simulink model "m03_model_for_state_feedback_design"  (R2021a)
settings: Solver=VariableStepAuto  StartTime=0.0  StopTime=10.0  MaxStep=1e-3  RelTol=1e-3
PreLoadFcn:
  | load feedforward_controller
  | load reduced_model
InitFcn:
  | load feedforward_controller
  | load reduced_model
values from neighbouring files (symbols this model uses):
  U0 = [0 0]    [linearization_data.mat]    (also in linearizedModel_Outputs.mat = [3.61873688012e-10 -3.90256021581e-22])
  Y0 = [0 0]    [linearization_data.mat]    (also in linearizedModel_Outputs.mat = [372.5 36.8372638482])
undefined symbols (not defined in the file or in its folder): X0_red
libraries: acolibjan22 x3
settings Model: Creator=e102261  LastModifiedBy=e102261
settings SolverCC: AlgebraicLoopSolver=TrustRegion
settings DataIOCC: SaveOutput=off  SignalLogging=off  DSMLogging=off  SaveTime=off  ReturnWorkspaceOutputs=off
settings DebuggingCC: ArithmeticOperatorsInVariantConditions=warning
settings SFSimCC: CustomCodeUndefinedFunction=UseInterfaceOnly

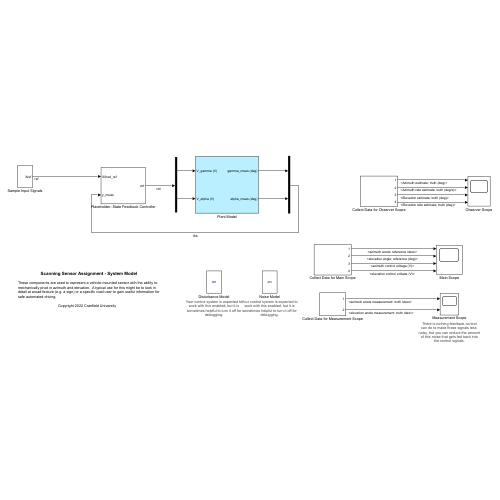
[thumbnail: Simulink's stored preview of the top-level diagram]
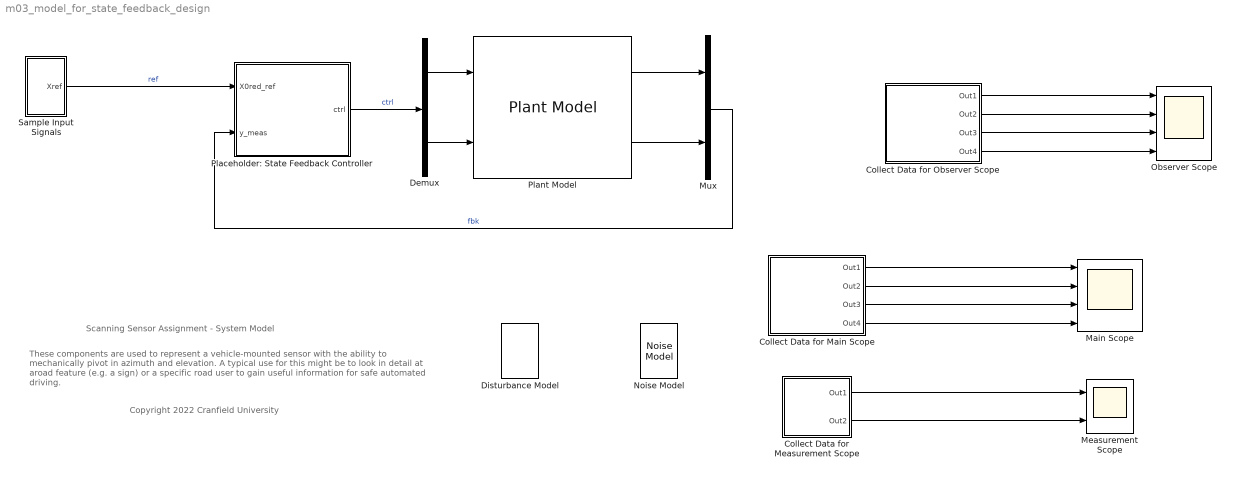
== system m03_model_for_state_feedback_design ==
  note: These components are used to represent a vehicle-mounted sensor with the ability to mechanically pivot in azimuth and elevation.  A typical use for this might be to look in
      | detail at aroad feature (e.g. a sign) or a specific road user to gain useful information for
      | safe automated driving.
  note: Scanning Sensor Assignment - System Model
  note: Copyright 2022 Cranfield University
  Collect Data for Main Scope : Subsystem
  Collect Data for Measurement Scope : Subsystem
  Collect Data for Observer Scope : Subsystem
  Demux : Demux  Outputs=2
  Disturbance Model : acolibjan22/Disturbance Model  EnabledState=on
      settings: AttributesFormatString=|
      | Your control system is expected to
      | work with this enabled, but it is
      | sometimes helpful to turn it off for
      | debugging.
  Main Scope : Scope  NumInputPorts=4
  Measurement Scope : Scope  NumInputPorts=2
      settings: AttributesFormatString=|
      | There is nothing feedback control
      | can do to make these signals less
      | noisy, but you can reduce the amount
      | of this noise that gets fed back into
      | the control signals.
  Mux : Mux  Inputs=2
  Noise Model : acolibjan22/Noise Model  EnabledState=on
      settings: AttributesFormatString=|
      | Your control system is expected to
      | work with this enabled, but it is
      | sometimes helpful to turn it off for
      | debugging.
  Observer Scope : Scope  NumInputPorts=4
  Placeholder: State Feedback Controller : Subsystem
  Plant Model : acolibjan22/Plant Model  X0=0
  Sample Input Signals : Subsystem
  wires:
  Plant Model/1 -> Mux/1
  Collect Data for Main Scope/1(Out1) -> Main Scope/1
  Collect Data for Main Scope/2(Out2) -> Main Scope/2
  Collect Data for Main Scope/3(Out3) -> Main Scope/3
  Collect Data for Main Scope/4(Out4) -> Main Scope/4
  Mux/1 -> Placeholder: State Feedback Controller/2(y_meas)  "fbk"
  Plant Model/2 -> Mux/2
  Demux/2 -> Plant Model/2
  Demux/1 -> Plant Model/1
  Collect Data for Measurement Scope/1(Out1) -> Measurement Scope/1
  Collect Data for Measurement Scope/2(Out2) -> Measurement Scope/2
  Placeholder: State Feedback Controller/1(ctrl) -> Demux/1  "ctrl"
  Collect Data for Observer Scope/1(Out1) -> Observer Scope/1
  Collect Data for Observer Scope/2(Out2) -> Observer Scope/2
  Collect Data for Observer Scope/3(Out3) -> Observer Scope/3
  Collect Data for Observer Scope/4(Out4) -> Observer Scope/4
  Sample Input Signals/1(Xref) -> Placeholder: State Feedback Controller/1(X0red_ref)  "ref"

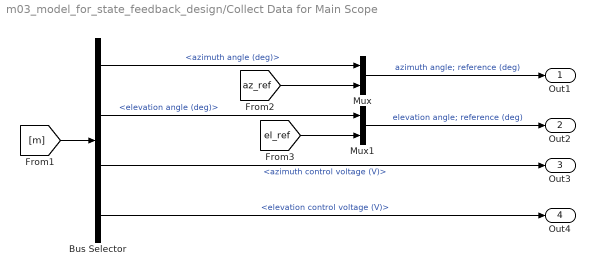
== system m03_model_for_state_feedback_design/Collect Data for Main Scope ==
  Bus Selector : BusSelector  OutputSignals=azimuth angle (deg),elevation angle (deg),azimuth control voltage (V),elevation control voltage (V)
  Mux : Mux  Inputs=2
  Mux1 : Mux  Inputs=2
  Out1 : Outport
  Out2 : Outport  Port=2
  Out3 : Outport  Port=3
  Out4 : Outport  Port=4
  wires:
  [m] -> Bus Selector/1
  Mux/1 -> Out1/1  "azimuth angle; reference (deg)"
  Bus Selector/1 -> Mux/1  "<azimuth angle (deg)>"
  [az_ref] -> Mux/2
  Bus Selector/2 -> Mux1/1  "<elevation angle (deg)>"
  [el_ref] -> Mux1/2
  Mux1/1 -> Out2/1  "elevation angle; reference (deg)"
  Bus Selector/3 -> Out3/1  "<azimuth control voltage (V)>"
  Bus Selector/4 -> Out4/1  "<elevation control voltage (V)>"

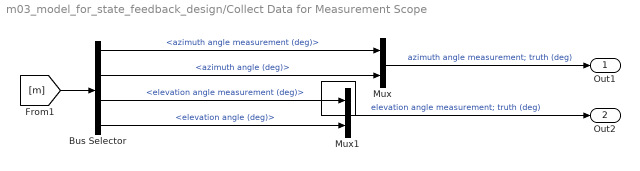
== system m03_model_for_state_feedback_design/Collect Data for Measurement Scope ==
  Bus Selector : BusSelector  OutputSignals=azimuth angle measurement (deg),azimuth angle (deg),elevation angle measurement (deg),elevation angle (deg)
  Mux : Mux  Inputs=2
  Mux1 : Mux  Inputs=2
  Out1 : Outport
  Out2 : Outport  Port=2
  wires:
  Mux1/1 -> Out2/1  "elevation angle measurement; truth (deg)"
  Bus Selector/4 -> Mux1/2  "<elevation angle (deg)>"
  Bus Selector/2 -> Mux/2  "<azimuth angle (deg)>"
  Mux/1 -> Out1/1  "azimuth angle measurement; truth (deg)"
  [m] -> Bus Selector/1
  Bus Selector/1 -> Mux/1  "<azimuth angle measurement (deg)>"
  Bus Selector/3 -> Mux1/1  "<elevation angle measurement (deg)>"

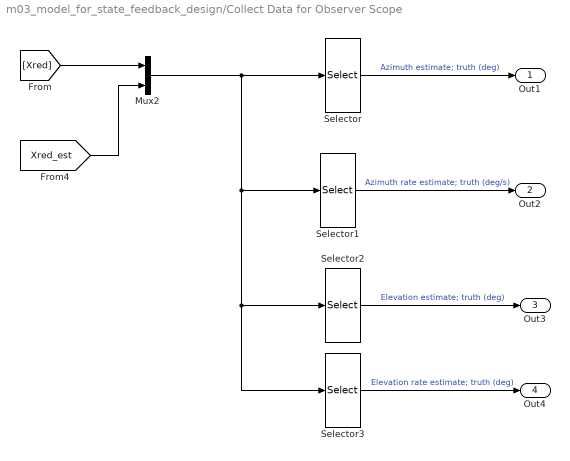
== system m03_model_for_state_feedback_design/Collect Data for Observer Scope ==
  Mux2 : Mux  Inputs=2
  Selector : Selector  InputPortWidth=8  IndexOptions=Index vector (dialog)  Indices=[1 5]  OutputSizes=1
  Selector1 : Selector  InputPortWidth=8  IndexOptions=Index vector (dialog)  Indices=[2 6]  OutputSizes=1
  Selector2 : Selector  InputPortWidth=8  IndexOptions=Index vector (dialog)  Indices=[3 7]  OutputSizes=1
  Selector3 : Selector  InputPortWidth=8  IndexOptions=Index vector (dialog)  Indices=[4 8]  OutputSizes=1
  Out1 : Outport
  Out2 : Outport  Port=2
  Out3 : Outport  Port=3
  Out4 : Outport  Port=4
  wires:
  [Xred] -> Mux2/1
  [Xred_est] -> Mux2/2
  Mux2/1 -> Selector3/1, Selector2/1, Selector1/1, Selector/1
  Selector/1 -> Out1/1  "Azimuth estimate; truth (deg)"
  Selector1/1 -> Out2/1  "Azimuth rate estimate; truth (deg/s)"
  Selector2/1 -> Out3/1  "Elevation estimate; truth (deg)"
  Selector3/1 -> Out4/1  "Elevation rate estimate; truth (deg)"

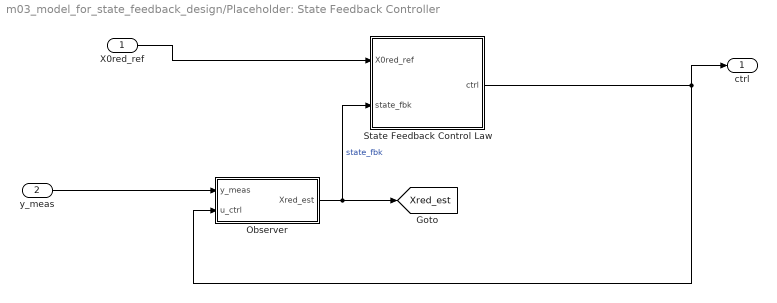
== system m03_model_for_state_feedback_design/Placeholder: State Feedback Controller ==
  X0red_ref : Inport  PortDimensions=4
  y_meas : Inport  Port=2  PortDimensions=2
  Observer : Subsystem
  State Feedback Control Law : Subsystem
  ctrl : Outport  PortDimensions=2
  tag scope: Xred_est=global
  wires:
  X0red_ref/1 -> State Feedback Control Law/1(X0red_ref)
  State Feedback Control Law/1(ctrl) -> ctrl/1, Observer/2(u_ctrl)
  Observer/1(Xred_est) -> [Xred_est], State Feedback Control Law/2(state_fbk)  "state_fbk"
  y_meas/1 -> Observer/1(y_meas)

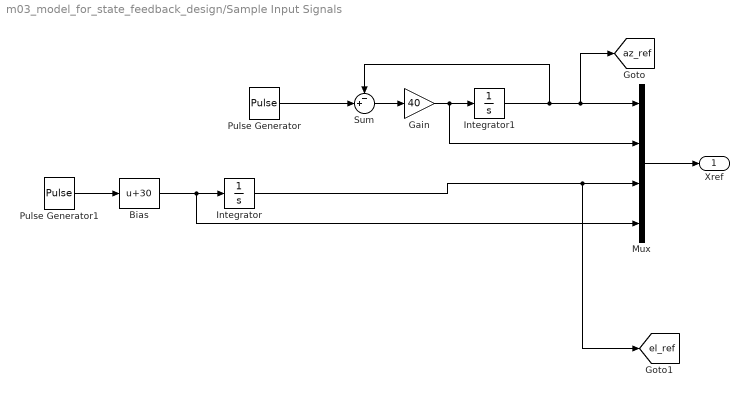
== system m03_model_for_state_feedback_design/Sample Input Signals ==
  Bias : Bias  Bias=30
  Gain : Gain  Gain=40
  Integrator : Integrator
  Integrator1 : Integrator
  Mux : Mux
  Pulse Generator : DiscretePulseGenerator  PulseType=Time based  Amplitude=35  Period=10  PulseWidth=50  PhaseDelay=1
  Pulse Generator1 : DiscretePulseGenerator  PulseType=Time based  Amplitude=-120/2  Period=4  PulseWidth=50  PhaseDelay=2
  Sum : Sum  Inputs=-+|
  Xref : Outport  PortDimensions=4
  tag scope: az_ref=global, el_ref=global
  wires:
  Pulse Generator/1 -> Sum/2
  Pulse Generator1/1 -> Bias/1
  Bias/1 -> Mux/4, Integrator/1
  Mux/1 -> Xref/1
  Gain/1 -> Mux/2, Integrator1/1
  Sum/1 -> Gain/1
  Integrator1/1 -> Sum/1, [az_ref], Mux/1
  Integrator/1 -> [el_ref], Mux/3

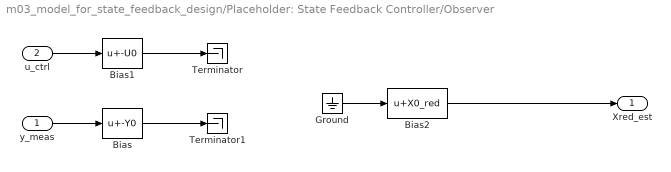
== system m03_model_for_state_feedback_design/Placeholder: State Feedback Controller/Observer ==
  y_meas : Inport  PortDimensions=2
  u_ctrl : Inport  Port=2
  Bias : Bias  Bias=-Y0
  Bias1 : Bias  Bias=-U0
  Bias2 : Bias  Bias=X0_red
  Ground : Ground
  Terminator : Terminator
  Terminator1 : Terminator
  Xred_est : Outport
  wires:
  y_meas/1 -> Bias/1
  u_ctrl/1 -> Bias1/1
  Bias1/1 -> Terminator/1
  Bias/1 -> Terminator1/1
  Ground/1 -> Bias2/1
  Bias2/1 -> Xred_est/1

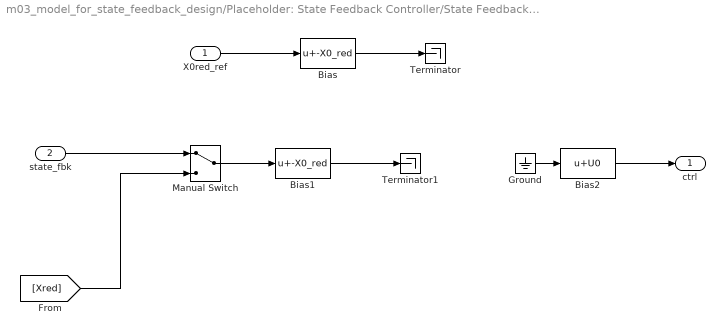
== system m03_model_for_state_feedback_design/Placeholder: State Feedback Controller/State Feedback Control Law ==
  X0red_ref : Inport
  state_fbk : Inport  Port=2
  Bias : Bias  Bias=-X0_red
  Bias1 : Bias  Bias=-X0_red
  Bias2 : Bias  Bias=U0
  Ground : Ground
  Manual Switch : ManualSwitch
      settings: AttributesFormatString=|
      | You can temporarily switch to
      | 'true values' so you can get a
      | state feedback controller working
      | separately from an observer.
  Terminator : Terminator
  Terminator1 : Terminator
  ctrl : Outport
  wires:
  state_fbk/1 -> Manual Switch/1
  X0red_ref/1 -> Bias/1
  Bias/1 -> Terminator/1
  Bias1/1 -> Terminator1/1
  Ground/1 -> Bias2/1
  Bias2/1 -> ctrl/1
  Manual Switch/1 -> Bias1/1
  [Xred] -> Manual Switch/2
